simulink model "LUPA_copy"  (R2024a)
settings: Solver=FixedStepAuto  StartTime=0.0  StopTime=Inf  FixedStep=Ts  RelTol=1e-3
PreLoadFcn:
  | addpath(genpath('utils'))
  | addpath(genpath('RLdata'))
  | load('modelWorkspace.mat')
  | load('referenceInit.mat')
  | ExcelGains = readtable(excelFile);  % read from excel spreadsheet gain values
  | ExcelGains = table2array(ExcelGains);
  | load('refSigs.mat')
  | 
  | z0 = 0;
  | v0 = 0;
  | 
  | Kp0 = 1000;
  | Ki0 = -300;
model workspace: external: MAT-File C:\Software\LUPA\Simulink\modelWorkspace.mat (data not in the file)
values from neighbouring files (symbols this model uses):
  C = 258.803991051052    (= 258.803991051)    [AOE_constants.m]
  CL = 13    [initLUPA.m]
  gainTstep = wavePeriod*10    (= 22.5)    [initLUPA.m]
  Kt = 7.86    [initLUPA.m]
  sprocketPitchRadius = 0.101854    [initLUPA.m]
  Ts = 0.001    [initLUPA.m]
undefined symbols (not defined in the file or in its folder): accX_mperssquared, accY_mperssquared, accZ_mperssquared, awasysstart, current_A, DClink_V, drawWire_m, drawWire_mpers, driveTemp_degC, eCATstate, IMUtemp_degC, Ki_max, Ki_min, Kp_max, Kp_min, led, linearPower_W, netForce_N, omegaPitch_radpers, omegaRoll_radpers, omegaYaw_radpers, opState, pos_cnts, pos_filt_rad, pos_rad, pow_W, sample, ShoreAI3, ShoreAI4, STOinterlock, T_s, tet, thetaPitch_deg, thetaRoll_deg, thetaYaw_deg, torque_Nm, vel_filt_radpers, vel_from_pos_radpers, vel_radpers
libraries: slrealtimeethercatlib x47, slrealtimeloglib x11, simulink x7, dspfdesign x4, spsSampleandHoldLib x3, slrealtimeutilitieslib x2, dspstat3 x2, rllib x1, slrealtimeptplib x1, slrealtimetgmanagement x1
settings Model: SimulationMode=external  ExtModeEnableFloating=off  Creator=HWRL user  LastModifiedBy=Wave User
settings SolverCC: ConcurrentTasks=on  PositivePriorityOrder=on
settings DataIOCC: ExternalInput=ds  LoadExternalInput=on
settings OptimizationCC: BlockReduction=off  OptimizeBlockIOStorage=off  ReuseModelBlockBuffer=off
settings DebuggingCC: TasksWithSamePriorityMsg=none  ParameterOverflowMsg=warning  ParameterPrecisionLossMsg=none  UnconnectedInputMsg=warning  UnconnectedOutputMsg=warning  UnconnectedLineMsg=warning
settings HardwareCC: ProdBitPerLong=64  ProdLongLongMode=on  ProdHWDeviceType=Intel->x86-64 (Linux 64)
settings ModelReferenceCC: EnableRefExpFcnMdlSchedulingChecks=on
settings SFSimCC: SimTargetLang=C++
settings RTWCC: Description=Speedgoat Real-Time Target Machine  SystemTargetFile=speedgoat.tlc  TemplateMakefile=slrealtime_default_tmf  RTWVerbose=off  Toolchain=Simulink Real-Time Toolchain  BuildConfiguration=Faster Runs  CodeExecutionProfiling=on  TargetLang=C++  GPUComputeCapability=3.5  DLArmComputeVersion=19.05
settings SimulinkRealTimeTargetCC: InstructionSetFMA=off  LogToMDFFile=off

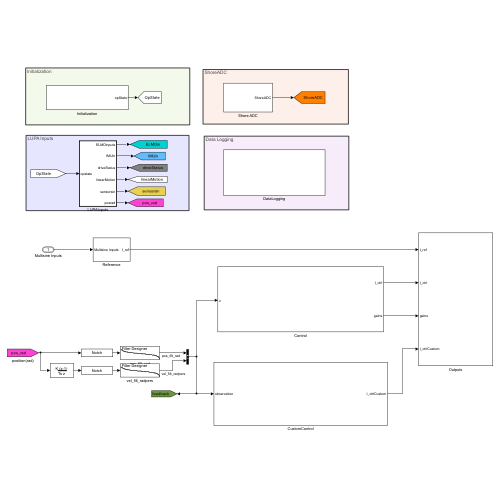
[thumbnail: Simulink's stored preview of the top-level diagram]
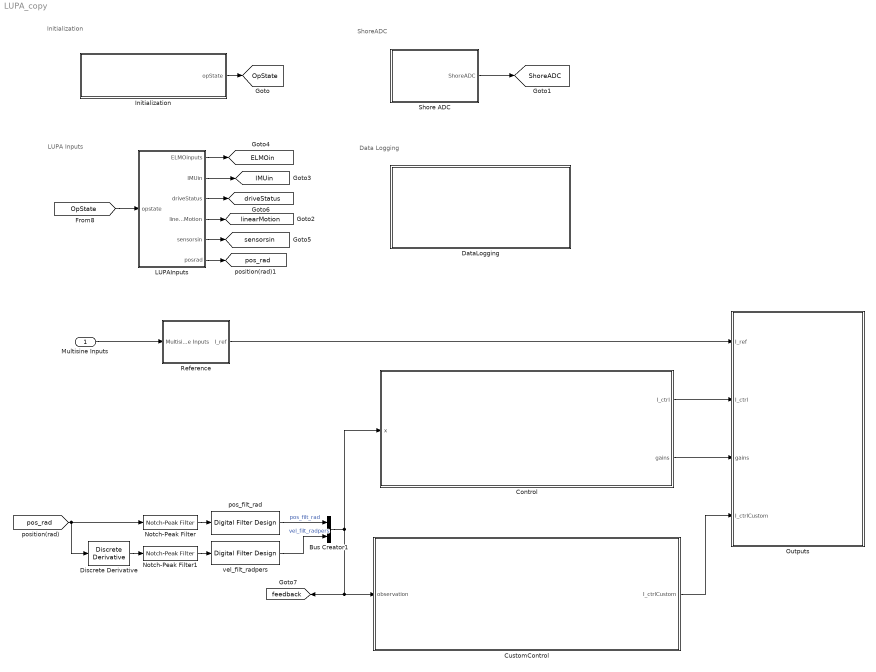
== system LUPA_copy ==
  note: Data Logging
  note: ShoreADC
  note: Initialization
  note: LUPA Inputs
  Multisine Inputs : Inport  OutDataTypeStr=Bus: refSigs
  Bus Creator1 : BusCreator  Inputs=pos_filt_rad,vel_filt_radpers
  Control : Subsystem
  CustomControl : Subsystem
  DataLogging : Subsystem
  Discrete Derivative : simulink/Discrete/Discrete Derivative  gainval=1.0  ICPrevScaledInput=0.0  OutMin=[]  OutMax=[]  OutDataType=fixdt(1, 16)  OutScaling=2^-10  DoSatur=off
  Initialization : Subsystem
  LUPAInputs : Subsystem  TreatAsAtomicUnit=on
  Notch-Peak Filter : dspfdesign/Notch-Peak Filter  Specification=Bandwidth and center frequency  BandwidthPort=off  Bandwidth=10  QualityFactorPort=off  QualityFactor=5  CenterFrequencyPort=off  CenterFrequency=50  BandwidthCoefficientPort=off  BandwidthCoefficient=0.72654  CenterFrequencyCoefficientPort=off  CenterFrequencyCoefficient=0  Output=Notch  SampleRateMode=Specify on dialog  SampleRate=1000  SimulateUsing=Code generation
  Notch-Peak Filter1 : dspfdesign/Notch-Peak Filter  Specification=Bandwidth and center frequency  BandwidthPort=off  Bandwidth=10  QualityFactorPort=off  QualityFactor=5  CenterFrequencyPort=off  CenterFrequency=50  BandwidthCoefficientPort=off  BandwidthCoefficient=0.72654  CenterFrequencyCoefficientPort=off  CenterFrequencyCoefficient=0  Output=Notch  SampleRateMode=Specify on dialog  SampleRate=1000  SimulateUsing=Code generation
  Outputs : Subsystem
  Reference : Subsystem
  Shore ADC : Subsystem
  pos_filt_rad : dspfdesign/Digital Filter Design  mwdsp_browser_bugfix_var=off
  vel_filt_radpers : dspfdesign/Digital Filter Design  mwdsp_browser_bugfix_var=off
  tag scope: ELMOin=global, IMUin=global, OpState=global, ShoreADC=global, driveStatus=global, feedback=global, linearMotion=global, pos_rad=global, sensorsin=global
  wires:
  Shore ADC/1(ShoreADC) -> [ShoreADC]
  Control/1(I_ctrl) -> Outputs/2(I_ctrl)
  Bus Creator1/1 -> Control/1(x), [feedback], CustomControl/1(observation)
  [pos_rad] -> Discrete Derivative/1, Notch-Peak Filter/1
  pos_filt_rad/1 -> Bus Creator1/1  "pos_filt_rad"
  Control/2(gains) -> Outputs/3(gains)
  CustomControl/1(I_ctrlCustom) -> Outputs/4(I_ctrlCustom)
  Reference/1(I_ref) -> Outputs/1(I_ref)
  Multisine Inputs/1 -> Reference/1(Multisine Inputs)
  Initialization/1(opState) -> [OpState]
  [OpState] -> LUPAInputs/1(opstate)
  LUPAInputs/1(ELMOinputs) -> [ELMOin]
  LUPAInputs/2(IMUin) -> [IMUin]
  LUPAInputs/3(driveStatus) -> [driveStatus]
  LUPAInputs/4(linearMotion) -> [linearMotion]
  LUPAInputs/5(sensorsin) -> [sensorsin]
  LUPAInputs/6(posrad) -> [pos_rad]
  Notch-Peak Filter/1 -> pos_filt_rad/1
  Notch-Peak Filter1/1 -> vel_filt_radpers/1
  vel_filt_radpers/1 -> Bus Creator1/2  "vel_filt_radpers"
  Discrete Derivative/1 -> Notch-Peak Filter1/1

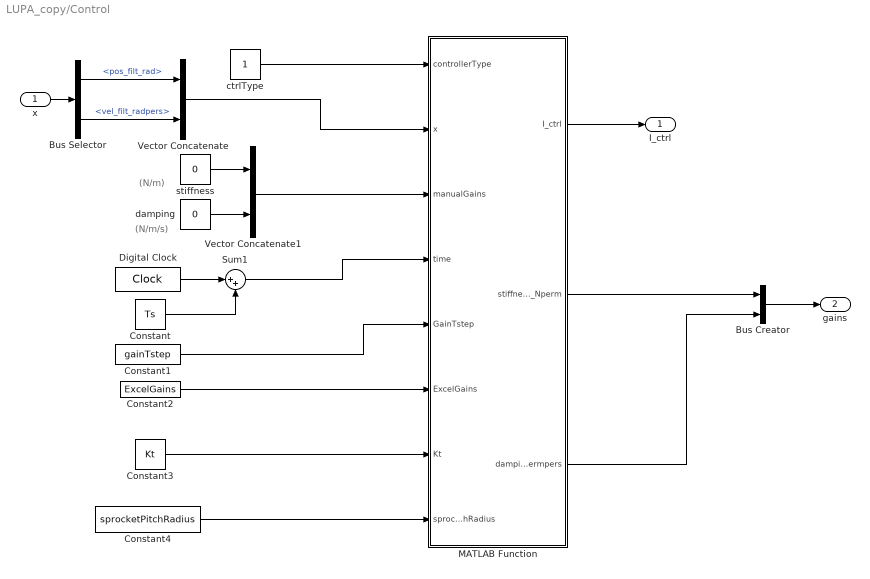
== system LUPA_copy/Control ==
  note: (N/m/s)
  note: (N/m)
  x : Inport
  Bus Creator : BusCreator  Inputs=2
  Bus Selector : BusSelector  OutputSignals=pos_filt_rad,vel_filt_radpers
  Constant : Constant  Value=Ts
  Constant1 : Constant  Value=gainTstep
  Constant2 : Constant  Value=ExcelGains  VectorParams1D=off
  Constant3 : Constant  Value=Kt
  Constant4 : Constant  Value=sprocketPitchRadius
  Digital Clock : DigitalClock  SampleTime=Ts
  MATLAB Function : MATLAB Function  TreatAsAtomicUnit=on
  Sum1 : Sum  Inputs=|++
  Vector Concatenate : Concatenate  Mode=Multidimensional array
  Vector Concatenate1 : Concatenate  Mode=Multidimensional array
  ctrlType : Constant
  damping : Constant  Value=0
  stiffness : Constant  Value=0
  I_ctrl : Outport
  gains : Outport  Port=2
  wires:
  stiffness/1 -> Vector Concatenate1/1
  Constant1/1 -> MATLAB Function/5(GainTstep)
  Constant/1 -> Sum1/2
  Vector Concatenate1/1 -> MATLAB Function/3(manualGains)
  Digital Clock/1 -> Sum1/1
  x/1 -> Bus Selector/1
  Sum1/1 -> MATLAB Function/4(time)
  Constant4/1 -> MATLAB Function/8(sprocketPitchRadius)
  damping/1 -> Vector Concatenate1/2
  Vector Concatenate/1 -> MATLAB Function/2(x)
  ctrlType/1 -> MATLAB Function/1(controllerType)
  Constant3/1 -> MATLAB Function/7(Kt)
  Constant2/1 -> MATLAB Function/6(ExcelGains)
  Bus Selector/1 -> Vector Concatenate/1  "<pos_filt_rad>"
  Bus Selector/2 -> Vector Concatenate/2  "<vel_filt_radpers>"
  MATLAB Function/1(I_ctrl) -> I_ctrl/1
  MATLAB Function/2(stiffness_Nperm) -> Bus Creator/1
  MATLAB Function/3(damping_Npermpers) -> Bus Creator/2
  Bus Creator/1 -> gains/1

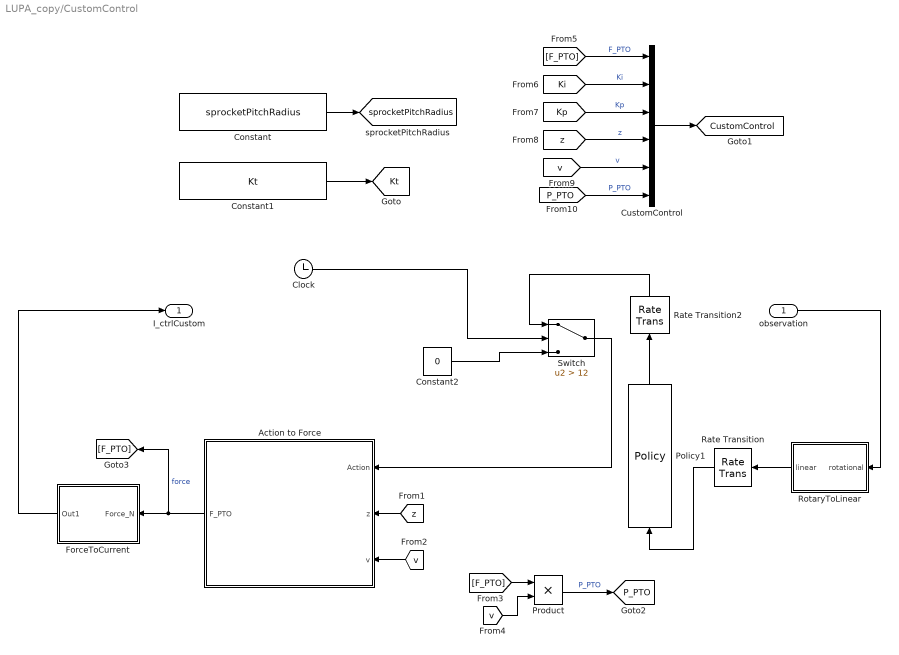
== system LUPA_copy/CustomControl ==
  observation : Inport
  Action to Force : Subsystem
  Clock : Clock
  Constant : Constant  Value=sprocketPitchRadius
  Constant1 : Constant  Value=Kt
  Constant2 : Constant  Value=0
  CustomControl : BusCreator  Inputs=6
  ForceToCurrent : Subsystem
  Policy1 : rllib/Policy  MATFile=blockAgentData.mat  PolicyParamsAsInput=off  PolicyParamsBusName=policy_param_bus  SimUsingCodegen=off
  Product : Product
  Rate Transition : RateTransition
  Rate Transition2 : RateTransition
  RotaryToLinear : Subsystem
  Switch : Switch  Criteria=u2 > Threshold  Threshold=12  SaturateOnIntegerOverflow=off  InputSameDT=off
  I_ctrlCustom : Outport
  tag scope: CustomControl=global, Kt=global, P_PTO=global, sprocketPitchRadius=global
  wires:
  Constant/1 -> [sprocketPitchRadius]
  Constant1/1 -> [Kt]
  ForceToCurrent/1(Out1) -> I_ctrlCustom/1
  [F_PTO] -> Product/1
  Action to Force/1(F_PTO) -> [F_PTO], ForceToCurrent/1(Force_N)  "force"
  [v] -> Product/2
  [v] -> Action to Force/3(v)
  [z] -> Action to Force/2(z)
  Product/1 -> [P_PTO]  "P_PTO"
  observation/1 -> RotaryToLinear/1(rotational)
  CustomControl/1 -> [CustomControl]
  [F_PTO] -> CustomControl/1  "F_PTO"
  [Ki] -> CustomControl/2  "Ki"
  [Kp] -> CustomControl/3  "Kp"
  [z] -> CustomControl/4  "z"
  [v] -> CustomControl/5  "v"
  [P_PTO] -> CustomControl/6  "P_PTO"
  Switch/1 -> Action to Force/1(Action)
  Constant2/1 -> Switch/3
  Clock/1 -> Switch/2
  RotaryToLinear/1(linear) -> Rate Transition/1
  Rate Transition/1 -> Policy1/1
  Policy1/1 -> Rate Transition2/1
  Rate Transition2/1 -> Switch/1

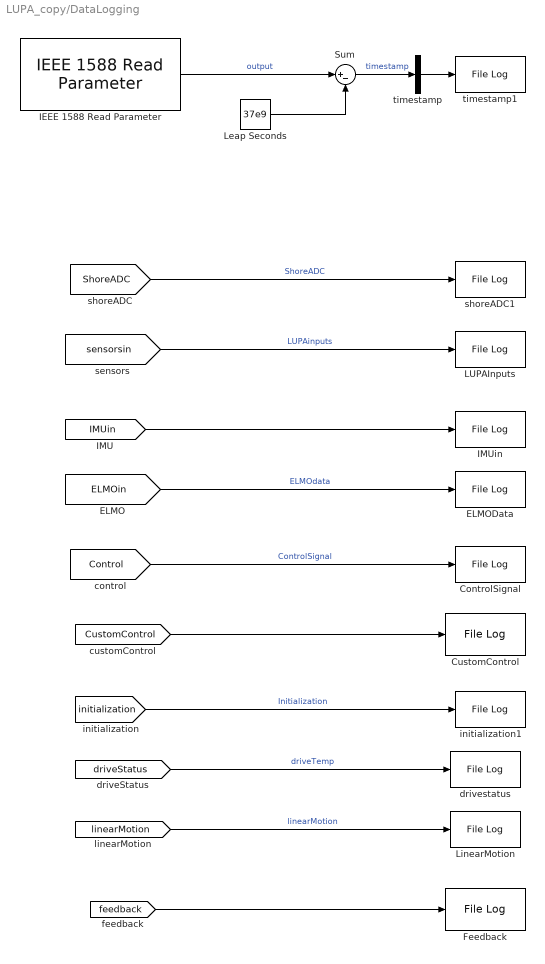
== system LUPA_copy/DataLogging ==
  ControlSignal : slrealtimeloglib/File Log  decimation=decimationLog  inputProcessing=Elements as channels (sample based)
  CustomControl : slrealtimeloglib/File Log  decimation=decimationLog  inputProcessing=Elements as channels (sample based)
  ELMOData : slrealtimeloglib/File Log  decimation=decimationLog  inputProcessing=Elements as channels (sample based)
  Feedback : slrealtimeloglib/File Log  decimation=1  inputProcessing=Elements as channels (sample based)
  IEEE 1588 Read Parameter : slrealtimeptplib/IEEE 1588 Read Parameter  Priority=1  ID=1  param=1. System time (nanosecond)  sample_time=Ts
  IMUin : slrealtimeloglib/File Log  decimation=decimationLog  inputProcessing=Elements as channels (sample based)
  LUPAInputs : slrealtimeloglib/File Log  decimation=decimationLog  inputProcessing=Elements as channels (sample based)
  Leap Seconds : Constant  Value=37e9  OutDataTypeStr=double
  LinearMotion : slrealtimeloglib/File Log  decimation=decimationLog  inputProcessing=Elements as channels (sample based)
  Sum : Sum  Inputs=|+-
  drivestatus : slrealtimeloglib/File Log  decimation=decimationLog  inputProcessing=Elements as channels (sample based)
  initialization1 : slrealtimeloglib/File Log  decimation=decimationLog  inputProcessing=Elements as channels (sample based)
  shoreADC1 : slrealtimeloglib/File Log  decimation=decimationLog  inputProcessing=Elements as channels (sample based)
  timestamp : BusCreator  Inputs=timestamp
  timestamp1 : slrealtimeloglib/File Log  decimation=decimationLog  inputProcessing=Elements as channels (sample based)
  wires:
  [ELMOin] -> ELMOData/1  "ELMOdata"
  [Control] -> ControlSignal/1  "ControlSignal"
  IEEE 1588 Read Parameter/1 -> Sum/1  "output"
  Sum/1 -> timestamp/1  "timestamp"
  timestamp/1 -> timestamp1/1
  Leap Seconds/1 -> Sum/2
  [initialization] -> initialization1/1  "Initialization"
  [sensorsin] -> LUPAInputs/1  "LUPAinputs"
  [IMUin] -> IMUin/1
  [driveStatus] -> drivestatus/1  "driveTemp"
  [ShoreADC] -> shoreADC1/1  "ShoreADC"
  [linearMotion] -> LinearMotion/1  "linearMotion"
  [feedback] -> Feedback/1
  [CustomControl] -> CustomControl/1

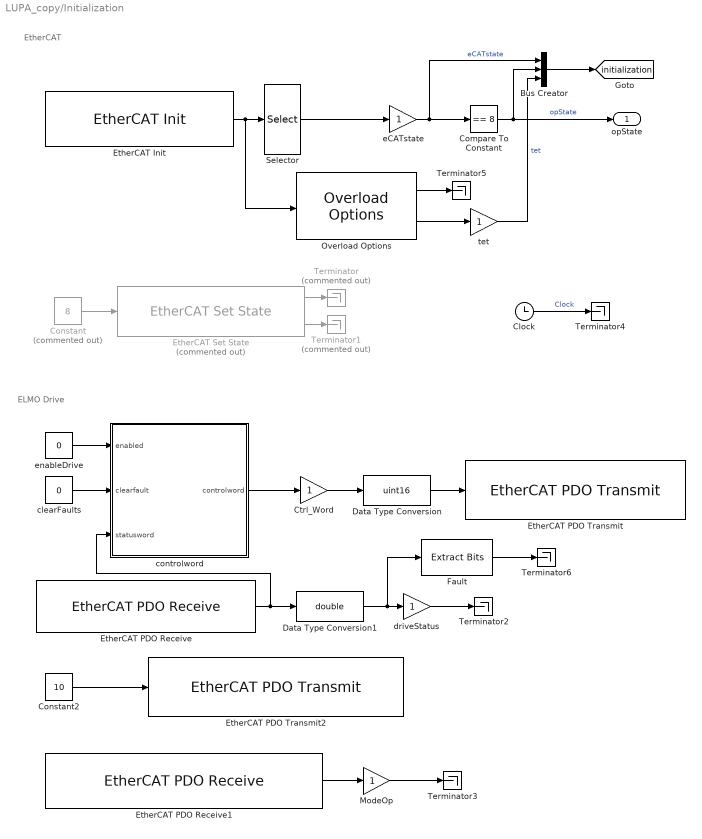
== system LUPA_copy/Initialization ==
  note: ELMO Drive
  note: EtherCAT
  Bus Creator : BusCreator  Inputs=eCATstate,opState,tet
  Clock : Clock
  Compare To Constant : simulink/Logic and Bit Operations/Compare To Constant  relop===  const=8  OutDataTypeStr=boolean
  Constant : Constant  Commented=on  Value=8  OutDataTypeStr=int32
  Constant2 : Constant  Value=10  OutDataTypeStr=int8
  Ctrl_Word : Gain
  Data Type Conversion : DataTypeConversion  OutDataTypeStr=uint16  SaturateOnIntegerOverflow=off  RndMeth=Floor
  Data Type Conversion1 : DataTypeConversion  OutDataTypeStr=double  SaturateOnIntegerOverflow=off  RndMeth=Floor
  EtherCAT Init : slrealtimeethercatlib/EtherCAT Init  Priority=0  config_file=C:\Software\LUPA\Simulink\EtherCAT\LUPA1kHz.xml  device_id=0  portnum=1  initstate=2  dctuning=0  enaDebug=0  logFile='c:\dbglog.txt'  sample_time=0.001000  DCMode=2
  EtherCAT PDO Receive : slrealtimeethercatlib/EtherCAT PDO Receive  Priority=2  sig_name=Drive 22 (Elmo Drive ).Inputs.Status word  sig_offset=2072  sig_type=uint16  type_size=16  sig_dim=1  device_id=0  sample_time=0.001000
  EtherCAT PDO Receive1 : slrealtimeethercatlib/EtherCAT PDO Receive  Priority=2  sig_name=Drive 22 (Elmo Drive ).Inputs_1.Mode of operation display  sig_offset=2088  sig_type=int8  type_size=8  sig_dim=1  device_id=0  sample_time=0.001000
  EtherCAT PDO Transmit : slrealtimeethercatlib/EtherCAT PDO Transmit  Priority=3  sig_name=Drive 22 (Elmo Drive ).Outputs.Control word  sig_offset=2072  sig_type=uint16  type_size=16  sig_dim=1  device_id=0  sample_time=0.001000
  EtherCAT PDO Transmit2 : slrealtimeethercatlib/EtherCAT PDO Transmit  Priority=3  sig_name=Drive 22 (Elmo Drive ).Outputs_1.Mode of operation  sig_offset=2088  sig_type=int8  type_size=8  sig_dim=1  device_id=0  sample_time=0.001000
  EtherCAT Set State : slrealtimeethercatlib/EtherCAT Set State  Commented=on  device_id=0  timeout=0  sample_time=0
  Fault : simulink/Logic and Bit Operations/Extract Bits  bitsToExtract=Range of bits  numBits=8  bitIdxRange=[3]  outScalingMode=Preserve fixed-point scaling
  ModeOp : Gain
  Overload Options : slrealtimetgmanagement/Overload Options  startupDur=1  startupDurSrc=Tunable Parameter  maxOverload=0  maxOverloadSrc=Tunable Parameter  TETFlag=on
  Selector : Selector  InputPortWidth=6  IndexOptions=Index vector (dialog)  Indices=2  OutputSizes=1
  Terminator : Terminator  Commented=on
  Terminator1 : Terminator  Commented=on
  Terminator{2..6} (5 alike) : Terminator
  clearFaults : Constant  Value=0
  controlword : MATLAB Function  TreatAsAtomicUnit=on
  driveStatus : Gain
  eCATstate : Gain  OutDataTypeStr=double
  enableDrive : Constant  Value=0
  tet : Gain  OutDataTypeStr=double
  opState : Outport
  tag scope: initialization=global
  wires:
  EtherCAT Init/1 -> Overload Options/1, Selector/1
  Selector/1 -> eCATstate/1
  Compare To Constant/1 -> opState/1, Bus Creator/2  "opState"
  EtherCAT Set State/1 -> Terminator/1
  EtherCAT Set State/2 -> Terminator1/1
  Constant/1 -> EtherCAT Set State/1
  EtherCAT PDO Receive/1 -> Data Type Conversion1/1, controlword/3(statusword)
  EtherCAT PDO Receive1/1 -> ModeOp/1
  Constant2/1 -> EtherCAT PDO Transmit2/1
  ModeOp/1 -> Terminator3/1
  Data Type Conversion1/1 -> Fault/1, driveStatus/1
  controlword/1(controlword) -> Ctrl_Word/1
  clearFaults/1 -> controlword/2(clearfault)
  Data Type Conversion/1 -> EtherCAT PDO Transmit/1
  driveStatus/1 -> Terminator2/1
  Ctrl_Word/1 -> Data Type Conversion/1
  enableDrive/1 -> controlword/1(enabled)
  eCATstate/1 -> Bus Creator/1, Compare To Constant/1  "eCATstate"
  Clock/1 -> Terminator4/1  "Clock"
  Bus Creator/1 -> [initialization]
  Overload Options/2 -> tet/1
  tet/1 -> Bus Creator/3  "tet"
  Overload Options/1 -> Terminator5/1
  Fault/1 -> Terminator6/1

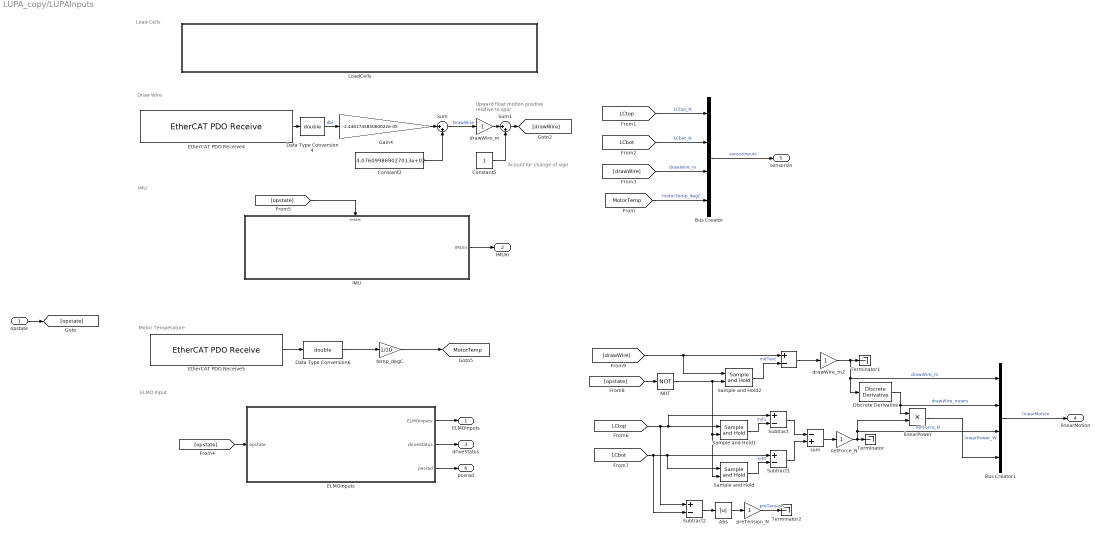
== system LUPA_copy/LUPAInputs ==
  note: Load Cells
  note: Acount for change of sign
  note: Upward float motion
      | positive relative to spar
  note: Motor Temperature
  note: ELMO Input
  note: Draw Wire
  note: IMU
  opstate : Inport
  " " : Sum  Inputs=+-
  Abs : Abs  SaturateOnIntegerOverflow=off
  Bus Creator : BusCreator  Inputs=4
  Bus Creator1 : BusCreator  Inputs=drawWire_m,drawWire_mpers,netForce_N,linearPower_W
  Constant2 : Constant  Value=4.076099869027013e+02
  Constant5 : Constant
  Data Type Conversion4 : DataTypeConversion  OutDataTypeStr=double  SaturateOnIntegerOverflow=off  RndMeth=Floor
  Data Type Conversion6 : DataTypeConversion  OutDataTypeStr=double  SaturateOnIntegerOverflow=off  RndMeth=Floor
  Discrete Derivative : simulink/Discrete/Discrete Derivative  gainval=1.0  ICPrevScaledInput=0.0  OutMin=[]  OutMax=[]  OutDataType=fixdt(1, 16)  OutScaling=2^-10  DoSatur=off
  ELMOInputs : Subsystem
  EtherCAT PDO Receive4 : slrealtimeethercatlib/EtherCAT PDO Receive  Priority=2  sig_name=Term 17 (EL5002).SSI Inputs Channel 1.Counter value  sig_offset=1000  sig_type=uint32  type_size=32  sig_dim=1  device_id=0  sample_time=0.001000
  EtherCAT PDO Receive5 : slrealtimeethercatlib/EtherCAT PDO Receive  Priority=2  sig_name=Term 21 (EL3202).RTD Inputs Channel 1.Value  sig_offset=1928  sig_type=int16  type_size=16  sig_dim=1  device_id=0  sample_time=0.001000
  Gain4 : Gain  Gain=-2.446174585060022e-05
  IMU : Subsystem  TreatAsAtomicUnit=on
  LoadCells : Subsystem
  NOT : Logic  Operator=NOT  IconShape=distinctive  AllPortsSameDT=off  OutDataTypeStr=boolean
  Sample and Hold : spsSampleandHoldLib/Sample and Hold  ic=0  Ts=Ts
  Sample and Hold1 : spsSampleandHoldLib/Sample and Hold  ic=1  Ts=Ts
  Sample and Hold2 : spsSampleandHoldLib/Sample and Hold  ic=0  Ts=Ts
  Subtract : Sum  Inputs=+-
  Subtract1 : Sum  Inputs=+-
  Subtract2 : Sum  Inputs=+-
  Sum : Sum  Inputs=|++
  Sum1 : Sum  Inputs=|++
  Terminator : Terminator
  Terminator1 : Terminator
  Terminator2 : Terminator
  drawWire_m : Gain  Gain=-1
  drawWire_m2 : Gain
  linearPower : Product
  netForce_N : Gain
  preTension_N : Gain
  sum : Sum  Inputs=-+
  temp_degC : Gain  Gain=1/10
  ELMOinputs : Outport
  IMUin : Outport  Port=2
  driveStatus : Outport  Port=3
  linearMotion : Outport  Port=4
  sensorsin : Outport  Port=5
  posrad : Outport  Port=6
  tag scope: MotorTemp=global
  wires:
  Data Type Conversion4/1 -> Gain4/1  "dbl"
  Gain4/1 -> Sum/1
  Constant2/1 -> Sum/2
  Sum/1 -> drawWire_m/1  "DrawWire"
  Bus Creator/1 -> sensorsin/1  "sensorInputs"
  Data Type Conversion6/1 -> temp_degC/1
  [MotorTemp] -> Bus Creator/4  "motorTemp_degC"
  [LCtop] -> Bus Creator/1  "LCtop_N"
  EtherCAT PDO Receive5/1 -> Data Type Conversion6/1
  temp_degC/1 -> [MotorTemp]
  [LCbot] -> Bus Creator/2  "LCbot_N"
  [drawWire] -> Bus Creator/3  "drawWire_m"
  EtherCAT PDO Receive4/1 -> Data Type Conversion4/1
  IMU/1(IMUin) -> IMUin/1
  [opstate] -> IMU/Enable
  sum/1 -> netForce_N/1
  Subtract1/1 -> sum/2
  Subtract/1 -> sum/1
  Sample and Hold/1 -> Subtract1/2  "init0"
  Sample and Hold1/1 -> Subtract/2  "init1"
  [LCtop] -> Subtract2/1, Subtract/1, Sample and Hold1/1
  [opstate] -> NOT/1
  Sample and Hold2/1 -> " "/2  "initTest"
  [drawWire] -> " "/1, Sample and Hold2/1
  " "/1 -> drawWire_m2/1
  [LCbot] -> Subtract2/2, Sample and Hold/1, Subtract1/1
  NOT/1 -> Sample and Hold2/2, Sample and Hold/2, Sample and Hold1/2
  netForce_N/1 -> Bus Creator1/3, linearPower/2, Terminator/1  "netForce_N"
  drawWire_m2/1 -> Bus Creator1/1, Discrete Derivative/1, Terminator1/1  "drawWire_m"
  drawWire_m/1 -> Sum1/1
  Sum1/1 -> [drawWire]
  Constant5/1 -> Sum1/2
  Discrete Derivative/1 -> Bus Creator1/2, linearPower/1  "drawWire_mpers"
  linearPower/1 -> Bus Creator1/4  "linearPower_W"
  Bus Creator1/1 -> linearMotion/1  "linearMotion"
  Subtract2/1 -> Abs/1
  Abs/1 -> preTension_N/1
  preTension_N/1 -> Terminator2/1  "preTension"
  opstate/1 -> [opstate]
  ELMOInputs/1(ELMOinputs) -> ELMOinputs/1
  ELMOInputs/2(driveStatus) -> driveStatus/1
  [opstate] -> ELMOInputs/1(opstate)
  ELMOInputs/3(posrad) -> posrad/1

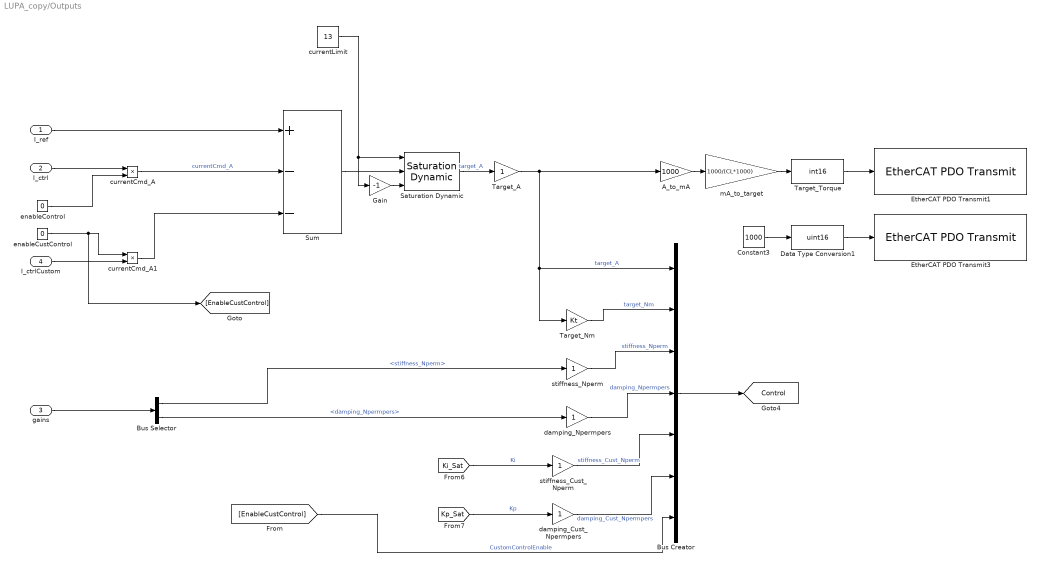
== system LUPA_copy/Outputs ==
  I_ref : Inport
  I_ctrl : Inport  Port=2
  gains : Inport  Port=3
  I_ctrlCustom : Inport  Port=4
  A_to_mA : Gain  Gain=1000
  Bus Creator : BusCreator  Inputs=7
  Bus Selector : BusSelector  OutputSignals=stiffness_Nperm,damping_Npermpers
  Constant3 : Constant  Value=1000  OutDataTypeStr=int16
  Data Type Conversion1 : DataTypeConversion  OutDataTypeStr=uint16  SaturateOnIntegerOverflow=off  RndMeth=Floor
  EtherCAT PDO Transmit1 : slrealtimeethercatlib/EtherCAT PDO Transmit  Priority=3  sig_name=Drive 22 (Elmo Drive ).Outputs_2.Target Torque  sig_offset=2104  sig_type=int16  type_size=16  sig_dim=1  device_id=0  sample_time=0.001000
  EtherCAT PDO Transmit3 : slrealtimeethercatlib/EtherCAT PDO Transmit  Priority=3  sig_name=Drive 22 (Elmo Drive ).Outputs_3.Max. Torque  sig_offset=2120  sig_type=uint16  type_size=16  sig_dim=1  device_id=0  sample_time=0.001000
  Gain : Gain  Gain=-1
  Saturation Dynamic : simulink/Discontinuities/Saturation Dynamic  OutMin=[]  OutMax=[]  OutDataTypeStr=Inherit: Same as second input  OutDataType=fixdt(1, 16)  OutScaling=2^-10  DoSatur=off
  Sum : Sum  Inputs=+--
  Target_A : Gain
  Target_Nm : Gain  Gain=Kt
  Target_Torque : DataTypeConversion  OutDataTypeStr=int16  SaturateOnIntegerOverflow=off  RndMeth=Floor
  currentCmd_A : Product
  currentCmd_A1 : Product
  currentLimit : Constant  Value=13
  damping_Cust_Npermpers : Gain
  damping_Npermpers : Gain
  enableControl : Constant  Value=0
  enableCustControl : Constant  Value=0
  mA_to_target : Gain  Gain=1000/(CL*1000)
  stiffness_Cust_Nperm : Gain
  stiffness_Nperm : Gain
  tag scope: Control=global
  wires:
  Constant3/1 -> Data Type Conversion1/1
  mA_to_target/1 -> Target_Torque/1
  Data Type Conversion1/1 -> EtherCAT PDO Transmit3/1
  Target_Torque/1 -> EtherCAT PDO Transmit1/1
  A_to_mA/1 -> mA_to_target/1
  currentCmd_A/1 -> Sum/2  "currentCmd_A"
  I_ref/1 -> Sum/1
  currentLimit/1 -> Gain/1, Saturation Dynamic/1
  enableControl/1 -> currentCmd_A/2
  I_ctrl/1 -> currentCmd_A/1
  Sum/1 -> Saturation Dynamic/2
  Gain/1 -> Saturation Dynamic/3
  Saturation Dynamic/1 -> Target_A/1  "target_A"
  Bus Selector/2 -> damping_Npermpers/1  "<damping_Npermpers>"
  Target_Nm/1 -> Bus Creator/2  "target_Nm"
  Bus Selector/1 -> stiffness_Nperm/1  "<stiffness_Nperm>"
  stiffness_Nperm/1 -> Bus Creator/3  "stiffness_Nperm"
  Bus Creator/1 -> [Control]
  Target_A/1 -> Target_Nm/1, Bus Creator/1, A_to_mA/1  "target_A"
  damping_Npermpers/1 -> Bus Creator/4  "damping_Npermpers"
  gains/1 -> Bus Selector/1
  currentCmd_A1/1 -> Sum/3
  I_ctrlCustom/1 -> currentCmd_A1/2
  enableCustControl/1 -> [EnableCustControl], currentCmd_A1/1
  [Ki_Sat] -> stiffness_Cust_Nperm/1  "Ki"
  [Kp_Sat] -> damping_Cust_Npermpers/1  "Kp"
  stiffness_Cust_Nperm/1 -> Bus Creator/5  "stiffness_Cust_Nperm"
  damping_Cust_Npermpers/1 -> Bus Creator/6  "damping_Cust_Npermpers"
  [EnableCustControl] -> Bus Creator/7  "CustomControlEnable"

== system LUPA_copy/Reference ==
  Multisine Inputs : Inport
  Bus Selector : BusSelector  OutputSignals=MS1,MS2,MS3
  Bus Selector1 : BusSelector  OutputSignals=ramps,sine,chirp,BLWN
  Multiport Switch : MultiPortSwitch  Inputs=8  SaturateOnIntegerOverflow=off  InputSameDT=off
  None : Constant  Value=0
  Subsystem Reference : Subsystem  ReferencedSubsystem=referenceSigs
  inputSwitch : Constant
  I_ref : Outport
  wires:
  inputSwitch/1 -> Multiport Switch/1
  Bus Selector/3 -> Multiport Switch/7  "<MS3>"
  Subsystem Reference/1 -> Bus Selector1/1
  Bus Selector/2 -> Multiport Switch/6  "<MS2>"
  Bus Selector1/2 -> Multiport Switch/4  "<sine>"
  Bus Selector1/4 -> Multiport Switch/9  "<BLWN>"
  Bus Selector1/3 -> Multiport Switch/8  "<chirp>"
  None/1 -> Multiport Switch/2
  Bus Selector/1 -> Multiport Switch/5  "<MS1>"
  Bus Selector1/1 -> Multiport Switch/3  "<ramps>"
  Multiport Switch/1 -> I_ref/1  "I_ref"
  Multisine Inputs/1 -> Bus Selector/1

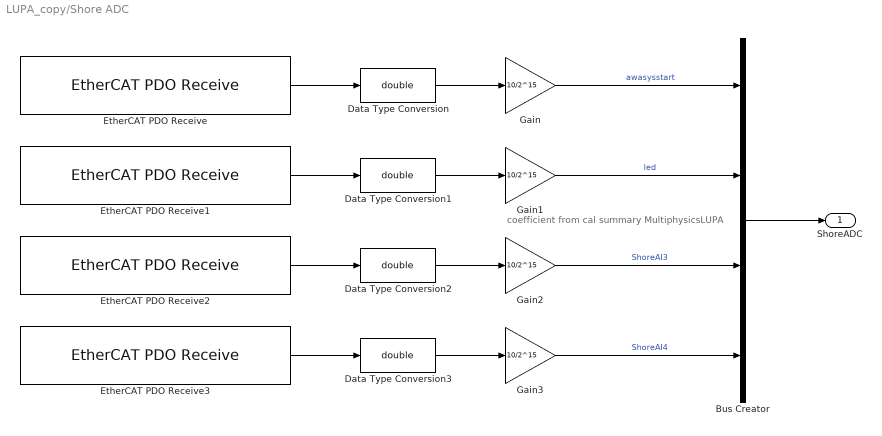
== system LUPA_copy/Shore ADC ==
  note: coefficient from cal summary MultiphysicsLUPA
  Bus Creator : BusCreator  Inputs=awasysstart,led,ShoreAI3,ShoreAI4
  Data Type Conversion{,1..3} (4 alike) : DataTypeConversion  OutDataTypeStr=double  SaturateOnIntegerOverflow=off  RndMeth=Floor
  EtherCAT PDO Receive : slrealtimeethercatlib/EtherCAT PDO Receive  Priority=2  sig_name=Term 15 (EL3104).AI Standard Channel 1.Value  sig_offset=872  sig_type=int16  type_size=16  sig_dim=1  device_id=0  sample_time=0.001000
  EtherCAT PDO Receive1 : slrealtimeethercatlib/EtherCAT PDO Receive  Priority=2  sig_name=Term 15 (EL3104).AI Standard Channel 2.Value  sig_offset=904  sig_type=int16  type_size=16  sig_dim=1  device_id=0  sample_time=0.001000
  EtherCAT PDO Receive2 : slrealtimeethercatlib/EtherCAT PDO Receive  Priority=2  sig_name=Term 15 (EL3104).AI Standard Channel 3.Value  sig_offset=936  sig_type=int16  type_size=16  sig_dim=1  device_id=0  sample_time=0.001000
  EtherCAT PDO Receive3 : slrealtimeethercatlib/EtherCAT PDO Receive  Priority=2  sig_name=Term 15 (EL3104).AI Standard Channel 4.Value  sig_offset=968  sig_type=int16  type_size=16  sig_dim=1  device_id=0  sample_time=0.001000
  Gain{,1..3} (4 alike) : Gain  Gain=10/2^15
  ShoreADC : Outport
  wires:
  EtherCAT PDO Receive/1 -> Data Type Conversion/1
  EtherCAT PDO Receive1/1 -> Data Type Conversion1/1
  EtherCAT PDO Receive2/1 -> Data Type Conversion2/1
  EtherCAT PDO Receive3/1 -> Data Type Conversion3/1
  Bus Creator/1 -> ShoreADC/1
  Data Type Conversion/1 -> Gain/1
  Data Type Conversion1/1 -> Gain1/1
  Data Type Conversion2/1 -> Gain2/1
  Data Type Conversion3/1 -> Gain3/1
  Gain/1 -> Bus Creator/1  "awasysstart"
  Gain3/1 -> Bus Creator/4  "ShoreAI4"
  Gain2/1 -> Bus Creator/3  "ShoreAI3"
  Gain1/1 -> Bus Creator/2  "led"

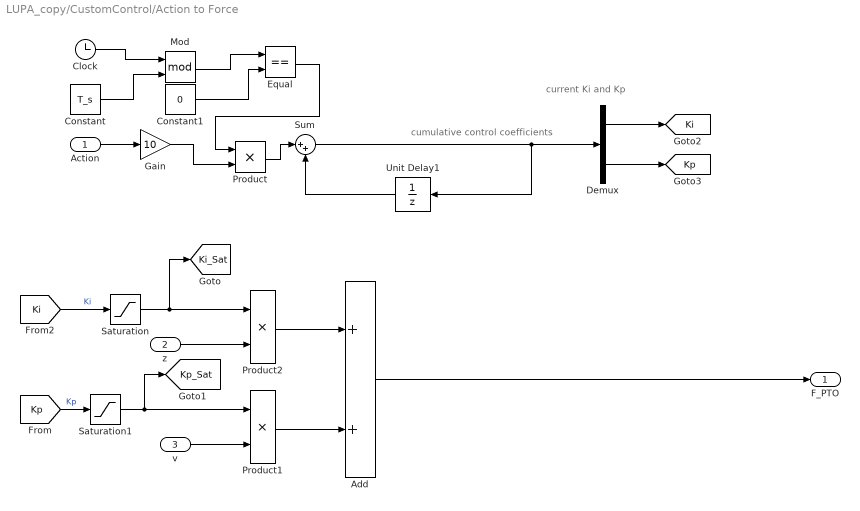
== system LUPA_copy/CustomControl/Action to Force ==
  note: cumulative control coefficients
  note: current Ki and Kp
  Action : Inport
  z : Inport  Port=2
  v : Inport  Port=3
  Add : Sum
  Clock : Clock
  Constant : Constant  Value=T_s
  Constant1 : Constant  Value=0
  Demux : Demux  Outputs=2
  Equal : RelationalOperator  Operator===  OutDataTypeStr=boolean  RndMeth=Simplest  InputSameDT=off
  Gain : Gain  Gain=10
  Mod : Math  Operator=mod
  Product : Product
  Product1 : Product
  Product2 : Product
  Saturation : Saturate  UpperLimit=Ki_max  LowerLimit=Ki_min
  Saturation1 : Saturate  UpperLimit=Kp_max  LowerLimit=Kp_min
  Sum : Sum  Inputs=|++
  Unit Delay1 : UnitDelay  InitialCondition=[Ki0;Kp0]  SampleTime=-1  HasFrameUpgradeWarning=on
  F_PTO : Outport
  tag scope: Ki=global, Ki_Sat=global, Kp=global, Kp_Sat=global
  wires:
  Demux/2 -> [Kp]
  Unit Delay1/1 -> Sum/2
  Action/1 -> Gain/1
  Sum/1 -> Unit Delay1/1, Demux/1
  Demux/1 -> [Ki]
  Product2/1 -> Add/1
  [Kp] -> Saturation1/1  "Kp"
  [Ki] -> Saturation/1  "Ki"
  Product1/1 -> Add/2
  Add/1 -> F_PTO/1
  z/1 -> Product2/2
  v/1 -> Product1/2
  Saturation/1 -> [Ki_Sat], Product2/1
  Saturation1/1 -> [Kp_Sat], Product1/1
  Clock/1 -> Mod/1
  Constant/1 -> Mod/2
  Mod/1 -> Equal/1
  Constant1/1 -> Equal/2
  Equal/1 -> Product/1
  Gain/1 -> Product/2
  Product/1 -> Sum/1

== system LUPA_copy/CustomControl/ForceToCurrent ==
  Force_N : Inport
  Divide : Product  Inputs=*/
  Product : Product
  Out1 : Outport
  wires:
  [sprocketPitchRadius] -> Product/2
  Product/1 -> Divide/1  "torque_Nm"
  Divide/1 -> Out1/1
  Force_N/1 -> Product/1
  [Kt] -> Divide/2

== system LUPA_copy/CustomControl/RotaryToLinear ==
  rotational : Inport
  Bus Creator : BusCreator  Inputs=2
  Bus Selector : BusSelector  OutputSignals=pos_filt_rad,vel_filt_radpers
  Product4 : Product
  Product5 : Product
  linear : Outport
  tag scope: v=global, z=global
  wires:
  Product5/1 -> Bus Creator/2, [v]  "vel_filt_mpers"
  Bus Selector/1 -> Product4/2  "<pos_filt_rad>"
  Bus Creator/1 -> linear/1
  rotational/1 -> Bus Selector/1
  Product4/1 -> Bus Creator/1, [z]  "pos_filt_m"
  [sprocketPitchRadius] -> Product5/2, Product4/1
  Bus Selector/2 -> Product5/1  "<vel_filt_radpers>"

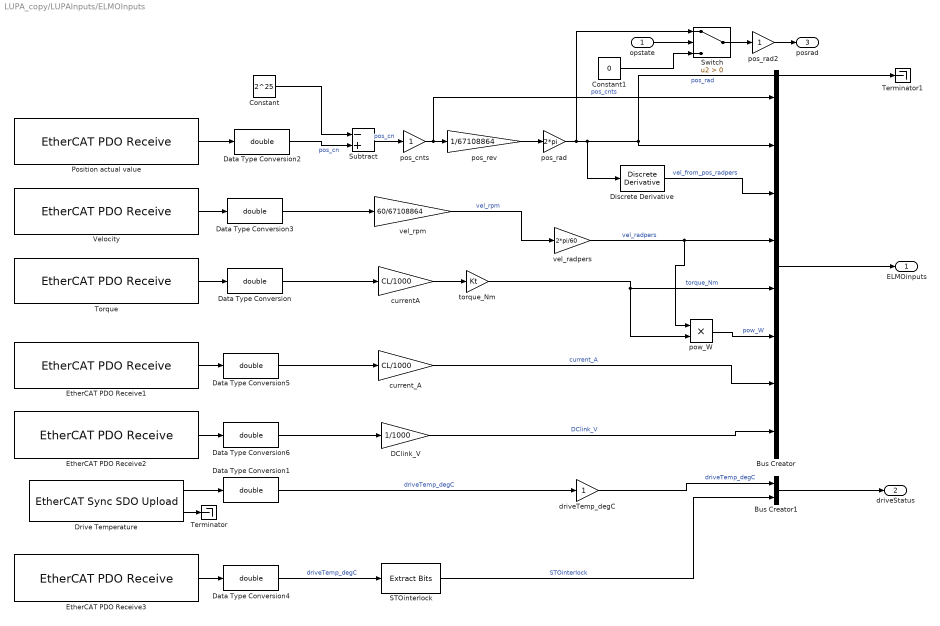
== system LUPA_copy/LUPAInputs/ELMOInputs ==
  opstate : Inport
  Bus Creator : BusCreator  Inputs=pos_cnts,pos_rad,vel_from_pos_radpers,vel_radpers,torque_Nm,pow_W,current_A,DClink_V
  Bus Creator1 : BusCreator  Inputs=driveTemp_degC,STOinterlock
  Constant : Constant  Value=2^25
  Constant1 : Constant  Value=0
  DClink_V : Gain  Gain=1/1000
  Data Type Conversion{,1..6} (7 alike) : DataTypeConversion  OutDataTypeStr=double  SaturateOnIntegerOverflow=off  RndMeth=Floor
  Discrete Derivative : simulink/Discrete/Discrete Derivative  gainval=1.0  ICPrevScaledInput=0.0  OutMin=[]  OutMax=[]  OutDataType=fixdt(1, 16)  OutScaling=2^-10  DoSatur=off
  Drive Temperature : slrealtimeethercatlib/EtherCAT Sync SDO Upload  index=0x22A3  subIndex=1  sig_type=int16  sig_dim=1  device_id=0  subdevice_name=Drive 22 (Elmo Drive )  sample_time=1  subdevice_addr=1009  selected_subdevice=Term 1 (EK1100)  timeout=500  subdevice_found=1  complete=0
  EtherCAT PDO Receive1 : slrealtimeethercatlib/EtherCAT PDO Receive  Priority=2  sig_name=Drive 22 (Elmo Drive ).Inputs_9.Current actual value  sig_offset=2312  sig_type=int16  type_size=16  sig_dim=1  device_id=0  sample_time=0.001000
  EtherCAT PDO Receive2 : slrealtimeethercatlib/EtherCAT PDO Receive  Priority=2  sig_name=Drive 22 (Elmo Drive ).Inputs_7.DC link circuit voltage  sig_offset=2248  sig_type=uint32  type_size=32  sig_dim=1  device_id=0  sample_time=0.001000
  EtherCAT PDO Receive3 : slrealtimeethercatlib/EtherCAT PDO Receive  Priority=2  sig_name=Drive 22 (Elmo Drive ).Inputs_8.Digital Inputs  sig_offset=2280  sig_type=uint32  type_size=32  sig_dim=1  device_id=0  sample_time=0.001000
  Position actual value : slrealtimeethercatlib/EtherCAT PDO Receive  Priority=2  sig_name=Drive 22 (Elmo Drive ).Inputs_3.Actual position [counts]  sig_offset=2136  sig_type=int32  type_size=32  sig_dim=1  device_id=0  sample_time=0.001000
  STOinterlock : simulink/Logic and Bit Operations/Extract Bits  bitsToExtract=Range of bits  numBits=8  bitIdxRange=[3]  outScalingMode=Preserve fixed-point scaling
  Subtract : Sum  Inputs=-+
  Switch : Switch  Criteria=u2 > Threshold  SaturateOnIntegerOverflow=off  InputSameDT=off
  Terminator : Terminator
  Terminator1 : Terminator
  Torque : slrealtimeethercatlib/EtherCAT PDO Receive  Priority=2  sig_name=Drive 22 (Elmo Drive ).Inputs_6.Torque actual value  sig_offset=2232  sig_type=int16  type_size=16  sig_dim=1  device_id=0  sample_time=0.001000
  Velocity : slrealtimeethercatlib/EtherCAT PDO Receive  Priority=2  sig_name=Drive 22 (Elmo Drive ).Inputs_5.Velocity sensor actual value [counts/sec]  sig_offset=2200  sig_type=int32  type_size=32  sig_dim=1  device_id=0  sample_time=0.001000
  currentA : Gain  Gain=CL/1000
  current_A : Gain  Gain=CL/1000
  driveTemp_degC : Gain
  pos_cnts : Gain
  pos_rad : Gain  Gain=2*pi
  pos_rad2 : Gain
  pos_rev : Gain  Gain=1/67108864
  pow_W : Product
  torque_Nm : Gain  Gain=Kt
  vel_radpers : Gain  Gain=2*pi/60
  vel_rpm : Gain  Gain=60/67108864
  ELMOinputs : Outport
  driveStatus : Outport  Port=2
  posrad : Outport  Port=3
  wires:
  EtherCAT PDO Receive1/1 -> Data Type Conversion5/1
  Data Type Conversion5/1 -> current_A/1
  EtherCAT PDO Receive2/1 -> Data Type Conversion6/1
  currentA/1 -> torque_Nm/1
  current_A/1 -> Bus Creator/7  "current_A"
  Data Type Conversion6/1 -> DClink_V/1
  pos_cnts/1 -> Bus Creator/1, pos_rev/1  "pos_cnts"
  pos_rad/1 -> Switch/1, Discrete Derivative/1, Terminator1/1, Bus Creator/2  "pos_rad"
  DClink_V/1 -> Bus Creator/8  "DClink_V"
  Velocity/1 -> Data Type Conversion3/1
  Data Type Conversion3/1 -> vel_rpm/1
  Subtract/1 -> pos_cnts/1  "pos_cn"
  vel_rpm/1 -> vel_radpers/1  "vel_rpm"
  torque_Nm/1 -> pow_W/2, Bus Creator/5  "torque_Nm"
  Position actual value/1 -> Data Type Conversion2/1
  Data Type Conversion/1 -> currentA/1
  Torque/1 -> Data Type Conversion/1
  pos_rev/1 -> pos_rad/1
  Bus Creator/1 -> ELMOinputs/1
  vel_radpers/1 -> pow_W/1, Bus Creator/4  "vel_radpers"
  Discrete Derivative/1 -> Bus Creator/3  "vel_from_pos_radpers"
  Drive Temperature/1 -> Data Type Conversion1/1
  Bus Creator1/1 -> driveStatus/1
  Drive Temperature/2 -> Terminator/1
  driveTemp_degC/1 -> Bus Creator1/1  "driveTemp_degC"
  Data Type Conversion1/1 -> driveTemp_degC/1  "driveTemp_degC"
  pow_W/1 -> Bus Creator/6  "pow_W"
  pos_rad2/1 -> posrad/1
  EtherCAT PDO Receive3/1 -> Data Type Conversion4/1
  Data Type Conversion4/1 -> STOinterlock/1  "driveTemp_degC"
  STOinterlock/1 -> Bus Creator1/2  "STOinterlock"
  Data Type Conversion2/1 -> Subtract/2  "pos_cn"
  Constant/1 -> Subtract/1
  Switch/1 -> pos_rad2/1
  opstate/1 -> Switch/2
  Constant1/1 -> Switch/3

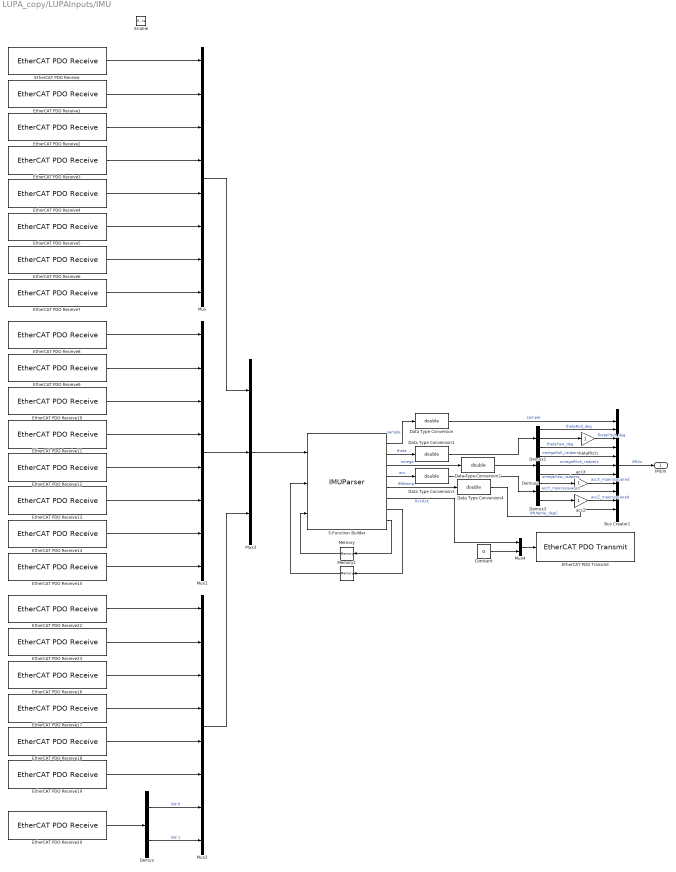
== system LUPA_copy/LUPAInputs/IMU ==
  Enable : EnablePort
  Bus Creator1 : BusCreator  Inputs=sample,thetaRoll_deg,thetaPitch_deg,thetaYaw_deg,omegaRoll_radpers,omegaPitch_radpers,omegaYaw_radpers,accX_mperssquared,accY_mperssquared,accZ_mperssquared,IMUtemp_degC
  Constant : Constant  Value=0  OutDataTypeStr=uint8
  Data Type Conversion{,1..4} (5 alike) : DataTypeConversion  OutDataTypeStr=double  SaturateOnIntegerOverflow=off  RndMeth=Floor
  Demux : Demux  Outputs=2
  Demux1 : Demux  Outputs=3
  Demux2 : Demux  Outputs=3
  Demux3 : Demux  Outputs=3
  EtherCAT PDO Receive : slrealtimeethercatlib/EtherCAT PDO Receive  Priority=2  sig_name=Term 18 (EL6001).COM Inputs.Data In 0  sig_offset=584  sig_type=uint8  type_size=8  sig_dim=1  device_id=0  sample_time=0.001000
  EtherCAT PDO Receive1 : slrealtimeethercatlib/EtherCAT PDO Receive  Priority=2  sig_name=Term 18 (EL6001).COM Inputs.Data In 1  sig_offset=592  sig_type=uint8  type_size=8  sig_dim=1  device_id=0  sample_time=0.001000
  EtherCAT PDO Receive10 : slrealtimeethercatlib/EtherCAT PDO Receive  Priority=2  sig_name=Term 18 (EL6001).COM Inputs.Data In 10  sig_offset=664  sig_type=uint8  type_size=8  sig_dim=1  device_id=0  sample_time=0.001000
  EtherCAT PDO Receive11 : slrealtimeethercatlib/EtherCAT PDO Receive  Priority=2  sig_name=Term 18 (EL6001).COM Inputs.Data In 11  sig_offset=672  sig_type=uint8  type_size=8  sig_dim=1  device_id=0  sample_time=0.001000
  EtherCAT PDO Receive12 : slrealtimeethercatlib/EtherCAT PDO Receive  Priority=2  sig_name=Term 18 (EL6001).COM Inputs.Data In 12  sig_offset=680  sig_type=uint8  type_size=8  sig_dim=1  device_id=0  sample_time=0.001000
  EtherCAT PDO Receive13 : slrealtimeethercatlib/EtherCAT PDO Receive  Priority=2  sig_name=Term 18 (EL6001).COM Inputs.Data In 13  sig_offset=688  sig_type=uint8  type_size=8  sig_dim=1  device_id=0  sample_time=0.001000
  EtherCAT PDO Receive14 : slrealtimeethercatlib/EtherCAT PDO Receive  Priority=2  sig_name=Term 18 (EL6001).COM Inputs.Data In 14  sig_offset=696  sig_type=uint8  type_size=8  sig_dim=1  device_id=0  sample_time=0.001000
  EtherCAT PDO Receive15 : slrealtimeethercatlib/EtherCAT PDO Receive  Priority=2  sig_name=Term 18 (EL6001).COM Inputs.Data In 15  sig_offset=704  sig_type=uint8  type_size=8  sig_dim=1  device_id=0  sample_time=0.001000
  EtherCAT PDO Receive16 : slrealtimeethercatlib/EtherCAT PDO Receive  Priority=2  sig_name=Term 18 (EL6001).COM Inputs.Data In 18  sig_offset=728  sig_type=uint8  type_size=8  sig_dim=1  device_id=0  sample_time=0.001000
  EtherCAT PDO Receive17 : slrealtimeethercatlib/EtherCAT PDO Receive  Priority=2  sig_name=Term 18 (EL6001).COM Inputs.Data In 19  sig_offset=736  sig_type=uint8  type_size=8  sig_dim=1  device_id=0  sample_time=0.001000
  EtherCAT PDO Receive18 : slrealtimeethercatlib/EtherCAT PDO Receive  Priority=2  sig_name=Term 18 (EL6001).COM Inputs.Data In 20  sig_offset=744  sig_type=uint8  type_size=8  sig_dim=1  device_id=0  sample_time=0.001000
  EtherCAT PDO Receive19 : slrealtimeethercatlib/EtherCAT PDO Receive  Priority=2  sig_name=Term 18 (EL6001).COM Inputs.Data In 21  sig_offset=752  sig_type=uint8  type_size=8  sig_dim=1  device_id=0  sample_time=0.001000
  EtherCAT PDO Receive2 : slrealtimeethercatlib/EtherCAT PDO Receive  Priority=2  sig_name=Term 18 (EL6001).COM Inputs.Data In 2  sig_offset=600  sig_type=uint8  type_size=8  sig_dim=1  device_id=0  sample_time=0.001000
  EtherCAT PDO Receive20 : slrealtimeethercatlib/EtherCAT PDO Receive  Priority=2  sig_name=Term 18 (EL6001).COM Inputs.Status  sig_offset=568  sig_type=uint8  type_size=8  sig_dim=2  device_id=0  sample_time=0.001000
  EtherCAT PDO Receive22 : slrealtimeethercatlib/EtherCAT PDO Receive  Priority=2  sig_name=Term 18 (EL6001).COM Inputs.Data In 16  sig_offset=712  sig_type=uint8  type_size=8  sig_dim=1  device_id=0  sample_time=0.001000
  EtherCAT PDO Receive23 : slrealtimeethercatlib/EtherCAT PDO Receive  Priority=2  sig_name=Term 18 (EL6001).COM Inputs.Data In 17  sig_offset=720  sig_type=uint8  type_size=8  sig_dim=1  device_id=0  sample_time=0.001000
  EtherCAT PDO Receive3 : slrealtimeethercatlib/EtherCAT PDO Receive  Priority=2  sig_name=Term 18 (EL6001).COM Inputs.Data In 3  sig_offset=608  sig_type=uint8  type_size=8  sig_dim=1  device_id=0  sample_time=0.001000
  EtherCAT PDO Receive4 : slrealtimeethercatlib/EtherCAT PDO Receive  Priority=2  sig_name=Term 18 (EL6001).COM Inputs.Data In 4  sig_offset=616  sig_type=uint8  type_size=8  sig_dim=1  device_id=0  sample_time=0.001000
  EtherCAT PDO Receive5 : slrealtimeethercatlib/EtherCAT PDO Receive  Priority=2  sig_name=Term 18 (EL6001).COM Inputs.Data In 5  sig_offset=624  sig_type=uint8  type_size=8  sig_dim=1  device_id=0  sample_time=0.001000
  EtherCAT PDO Receive6 : slrealtimeethercatlib/EtherCAT PDO Receive  Priority=2  sig_name=Term 18 (EL6001).COM Inputs.Data In 6  sig_offset=632  sig_type=uint8  type_size=8  sig_dim=1  device_id=0  sample_time=0.001000
  EtherCAT PDO Receive7 : slrealtimeethercatlib/EtherCAT PDO Receive  Priority=2  sig_name=Term 18 (EL6001).COM Inputs.Data In 7  sig_offset=640  sig_type=uint8  type_size=8  sig_dim=1  device_id=0  sample_time=0.001000
  EtherCAT PDO Receive8 : slrealtimeethercatlib/EtherCAT PDO Receive  Priority=2  sig_name=Term 18 (EL6001).COM Inputs.Data In 8  sig_offset=648  sig_type=uint8  type_size=8  sig_dim=1  device_id=0  sample_time=0.001000
  EtherCAT PDO Receive9 : slrealtimeethercatlib/EtherCAT PDO Receive  Priority=2  sig_name=Term 18 (EL6001).COM Inputs.Data In 9  sig_offset=656  sig_type=uint8  type_size=8  sig_dim=1  device_id=0  sample_time=0.001000
  EtherCAT PDO Transmit : slrealtimeethercatlib/EtherCAT PDO Transmit  Priority=3  sig_name=Term 18 (EL6001).COM Outputs.Ctrl  sig_offset=568  sig_type=uint8  type_size=8  sig_dim=2  device_id=0  sample_time=0.001000
  Memory : Memory
  Memory1 : Memory  InitialCondition=[zeros(4,1);-1;zeros(11,1)]
  Mux : Mux  Inputs=8
  Mux1 : Mux  Inputs=8
  Mux2 : Mux  Inputs=8
  Mux3 : Mux  Inputs=3
  Mux4 : Mux  Inputs=2
  S-Function Builder : S-Function  FunctionName=IMUParser  SFunctionModules=IMUParser_wrapper.cpp  SFunctionDeploymentMode=off  EnableBusSupport=off  mask(S-Function Builder){}
      mask help: Simulink:masks:SFunctionBuilder_MD
      mask init:
      | val = [[.9  0.75 0.75 1 1 .9 .9 1]',[1 1 0.75 0.75 .9 .9 1 .9]'];try , sys = get_param(gcb,'SfunBuilderFcnName');if isempty(sys), sys = get_param(gcb,'FunctionName'); end,catch, sys = get_param(gcb,'FunctionName'); end
      settings: CopyFcn=set_param(gcbh,'LinkStatus','none')  OpenFcn=sfunctionwizard(gcbh)
      mask Display:
      | plot(val(:,1),val(:,2))
      | disp(sys)
      | port_label('input',1,sprintf('%s', 'u0'),'interpreter','tex')
      | port_label('input',2,sprintf('%s', 'mem'),'interpreter','tex')
      | port_label('input',3,sprintf('%s', 'buffin'),'interpreter','tex')
      | port_label('output',1,sprintf('%s', 'samp'),'interpreter','tex')
      | port_label('output',2,sprintf('%s', 'theta'),'interpreter','tex')
      | port_label('output',3,sprintf('%s', 'omega'),'interpreter','tex')
      | port_label('output',4,sprintf('%s', 'acc'),'interpreter','tex')
      | port_label('output',5,sprintf('%s', 'IMUtemp'),'interpreter','tex')
      | port_label('output',6,sprintf('%s', 'RcvAck'),'interpreter','tex')
      | port_label('output',7,sprintf('%s', 'memout'),'interpreter','tex')
      | port_label('output',8,sprintf('%s', 'buffer'),'interpreter','tex')
  accX : Gain
  accZ : Gain
  thetaPitch : Gain
  IMUin : Outport
  wires:
  EtherCAT PDO Receive/1 -> Mux/1
  EtherCAT PDO Receive1/1 -> Mux/2
  EtherCAT PDO Receive2/1 -> Mux/3
  EtherCAT PDO Receive3/1 -> Mux/4
  EtherCAT PDO Receive4/1 -> Mux/5
  EtherCAT PDO Receive5/1 -> Mux/6
  EtherCAT PDO Receive6/1 -> Mux/7
  EtherCAT PDO Receive7/1 -> Mux/8
  EtherCAT PDO Receive15/1 -> Mux1/8
  EtherCAT PDO Receive14/1 -> Mux1/7
  EtherCAT PDO Receive13/1 -> Mux1/6
  EtherCAT PDO Receive12/1 -> Mux1/5
  EtherCAT PDO Receive11/1 -> Mux1/4
  EtherCAT PDO Receive10/1 -> Mux1/3
  EtherCAT PDO Receive9/1 -> Mux1/2
  EtherCAT PDO Receive8/1 -> Mux1/1
  EtherCAT PDO Receive22/1 -> Mux2/1
  EtherCAT PDO Receive23/1 -> Mux2/2
  EtherCAT PDO Receive16/1 -> Mux2/3
  EtherCAT PDO Receive17/1 -> Mux2/4
  EtherCAT PDO Receive18/1 -> Mux2/5
  EtherCAT PDO Receive19/1 -> Mux2/6
  Demux/1 -> Mux2/7  "SW.0"
  Demux/2 -> Mux2/8  "SW.1"
  EtherCAT PDO Receive20/1 -> Demux/1
  Mux1/1 -> Mux3/2
  Mux/1 -> Mux3/1
  Mux2/1 -> Mux3/3
  Mux3/1 -> S-Function Builder/1
  S-Function Builder/7 -> Memory1/1
  Memory1/1 -> S-Function Builder/2
  S-Function Builder/8 -> Memory/1
  Memory/1 -> S-Function Builder/3
  S-Function Builder/6 -> Mux4/1  "RcvAck"
  Constant/1 -> Mux4/2
  Mux4/1 -> EtherCAT PDO Transmit/1
  S-Function Builder/2 -> Data Type Conversion1/1  "theta"
  S-Function Builder/3 -> Data Type Conversion2/1  "omega"
  S-Function Builder/4 -> Data Type Conversion3/1  "acc"
  S-Function Builder/1 -> Data Type Conversion/1  "sample"
  Demux1/1 -> Bus Creator1/2  "thetaRoll_deg"
  Demux1/2 -> thetaPitch/1
  Demux1/3 -> Bus Creator1/4  "thetaYaw_deg"
  Demux2/3 -> Bus Creator1/7  "omegaYaw_radpers"
  Demux2/2 -> Bus Creator1/6  "omegaPitch_radpers"
  Demux2/1 -> Bus Creator1/5  "omegaRoll_radpers"
  Demux3/1 -> accX/1
  Demux3/2 -> Bus Creator1/9  "accY_mperssquared"
  Demux3/3 -> accZ/1
  S-Function Builder/5 -> Data Type Conversion4/1  "IMUtemp"
  Bus Creator1/1 -> IMUin/1  "IMUin"
  thetaPitch/1 -> Bus Creator1/3  "thetaPitch_deg"
  accX/1 -> Bus Creator1/8  "accX_mperssquared"
  accZ/1 -> Bus Creator1/10  "accZ_mperssquared"
  Data Type Conversion/1 -> Bus Creator1/1  "sample"
  Data Type Conversion1/1 -> Demux1/1
  Data Type Conversion2/1 -> Demux2/1
  Data Type Conversion3/1 -> Demux3/1
  Data Type Conversion4/1 -> Bus Creator1/11  "IMUtemp_degC"

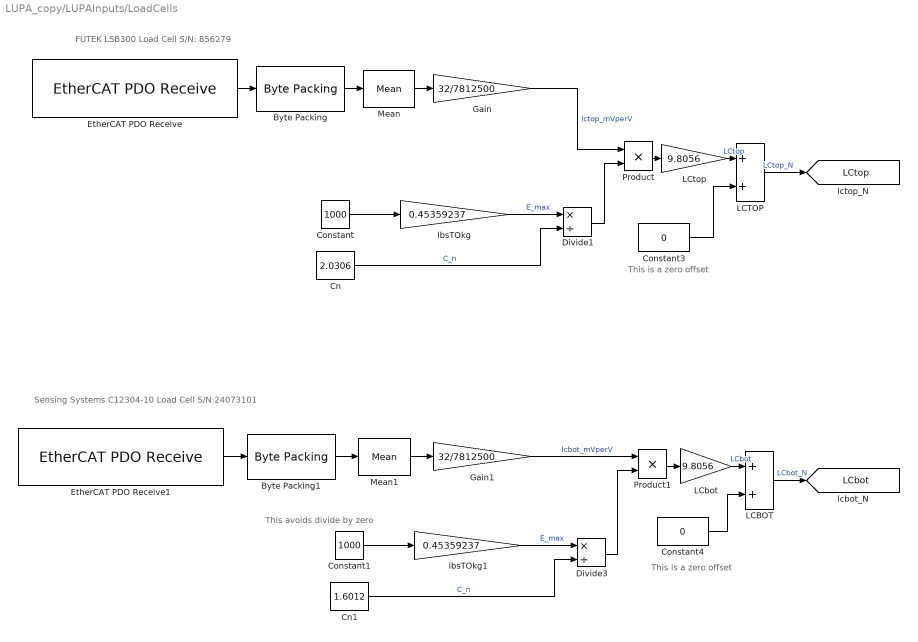
== system LUPA_copy/LUPAInputs/LoadCells ==
  note: This is a zero offset
  note: FUTEK LSB300 Load Cell S/N: 856279
  note: Sensing Systems C12304-10 Load Cell S/N:24073101
  note: This avoids divide by zero
  note: This is a zero offset
  Byte Packing : slrealtimeutilitieslib/Byte Packing  MaskPackedDataType=int32  MaskUnpackedDataTypes={'uint8'}  MaskAlignment=1
  Byte Packing1 : slrealtimeutilitieslib/Byte Packing  MaskPackedDataType=int32  MaskUnpackedDataTypes={'uint8'}  MaskAlignment=1
  Cn : Constant  Value=2.0306
  Cn1 : Constant  Value=1.6012
  Constant : Constant  Value=1000
  Constant1 : Constant  Value=1000
  Constant3 : Constant  Value=0
  Constant4 : Constant  Value=0
  Divide1 : Product  Inputs=*/
  Divide3 : Product  Inputs=*/
  EtherCAT PDO Receive : slrealtimeethercatlib/EtherCAT PDO Receive  Priority=2  sig_name=Term 20 (EL3751).PAI Samples 10.Samples  sig_offset=1528  sig_type=uint8  type_size=8  sig_dim=40  device_id=0  sample_time=0.001000
  EtherCAT PDO Receive1 : slrealtimeethercatlib/EtherCAT PDO Receive  Priority=2  sig_name=Term 19 (EL3751).PAI Samples 10.Samples  sig_offset=1112  sig_type=uint8  type_size=8  sig_dim=40  device_id=0  sample_time=0.001000
  Gain : Gain  Gain=32/7812500
  Gain1 : Gain  Gain=32/7812500
  LCBOT : Sum
  LCTOP : Sum
  LCbot : Gain  Gain=9.8056
  LCtop : Gain  Gain=9.8056
  Mean : dspstat3/Mean  run=off  InputProcessing=Columns as channels (frame based)  reset_popup=None  directionMode=Each column  dimension=1  roiEnable=off  roiType=Rectangles  roiPortion=Entire ROI  roiOutput=Individual statistics for each ROI  roiFlag=off  roundingMode=Floor  overflowMode=off  outputDataTypeStr=Inherit: Same as accumulator  outputMin=[]  outputMax=[]  outputLastDataTypeStr=Inherit: Same as accumulator
  Mean1 : dspstat3/Mean  run=off  InputProcessing=Columns as channels (frame based)  reset_popup=None  directionMode=Each column  dimension=1  roiEnable=off  roiType=Rectangles  roiPortion=Entire ROI  roiOutput=Individual statistics for each ROI  roiFlag=off  roundingMode=Floor  overflowMode=off  outputDataTypeStr=Inherit: Same as accumulator  outputMin=[]  outputMax=[]  outputLastDataTypeStr=Inherit: Same as accumulator
  Product : Product
  Product1 : Product
  lbsTOkg : Gain  Gain=0.45359237
  lbsTOkg1 : Gain  Gain=0.45359237
  tag scope: LCbot=global, LCtop=global
  wires:
  Constant/1 -> lbsTOkg/1
  Gain1/1 -> Product1/1  "lcbot_mVperV"
  Constant3/1 -> LCTOP/2
  Byte Packing1/1 -> Mean1/1
  LCTOP/1 -> [LCtop]  "LCtop_N"
  EtherCAT PDO Receive1/1 -> Byte Packing1/1
  Product1/1 -> LCbot/1
  LCBOT/1 -> [LCbot]  "LCbot_N"
  Gain/1 -> Product/1  "lctop_mVperV"
  Divide3/1 -> Product1/2
  Mean1/1 -> Gain1/1
  Divide1/1 -> Product/2
  Byte Packing/1 -> Mean/1
  lbsTOkg/1 -> Divide1/1  "E_max"
  LCbot/1 -> LCBOT/1  "LCbot"
  Mean/1 -> Gain/1
  EtherCAT PDO Receive/1 -> Byte Packing/1
  lbsTOkg1/1 -> Divide3/1  "E_max"
  Product/1 -> LCtop/1
  Cn1/1 -> Divide3/2  "C_n"
  Constant4/1 -> LCBOT/2
  Cn/1 -> Divide1/2  "C_n"
  Constant1/1 -> lbsTOkg1/1
  LCtop/1 -> LCTOP/1  "LCtop"

== matlab function LUPA_copy/Control/MATLAB Function ==
  data: controllerType input; x input; I_ctrl output; manualGains input; stiffness_Nperm output; time input; GainTstep input; ExcelGains input; Kt input; sprocketPitchRadius input; damping_Npermpers output
function [I_ctrl, stiffness_Nperm, damping_Npermpers] = fcn(controllerType, x, manualGains,time,GainTstep,ExcelGains, Kt, sprocketPitchRadius)
% gain format [positionProportional, velocityProportional]
% x format [theta; omega]

I_ctrl = 0;
gainMat = zeros(1,2);

if controllerType == 1

    B = sprocketPitchRadius^2 / Kt * manualGains' * x;
    stiffness_Nperm = manualGains(1);
    damping_Npermpers = manualGains(2);
elseif controllerType == 2
    idx = ceil(time./GainTstep); % Find index of current gain step
    while idx > length(ExcelGains(:,1))
        idx = idx-length(ExcelGains(:,1));
    end
    gainMat(1,1) = ExcelGains(idx,1);
    gainMat(1,2) = ExcelGains(idx,2);
    B = sprocketPitchRadius^2 / Kt * gainMat* x;
    stiffness_Nperm = gainMat(1,1);
    damping_Npermpers = gainMat(1,2);
else
    B = 0;
    stiffness_Nperm = 0;
    damping_Npermpers = 0;
end

I_ctrl = B;

== matlab function LUPA_copy/Initialization/controlword ==
  data: enabled input; clearfault input; statusword input; controlword output
function controlword = fcn(enabled, clearfault, statusword)

bitstatus = bitget(statusword,1:16);

if ~clearfault
    if enabled
        if bitstatus(1) == 0 % Ready to switch on not ready
            controlword = 6; % command ready switch on
        elseif ~bitstatus(2) % switched not yet on
            controlword = 7; % command switch on
        elseif ~bitstatus(3) % operation not yet enabled
            controlword = 15; % command enable
        else
            controlword = 15; % maintain enabled state
        end
    else
        controlword = 4; % command disabled
    end
else
    controlword = 128; % command clear faults
end
